simulink model "oUmControlador1"  (R2018a)
settings: Solver=VariableStepAuto  StartTime=0.0  StopTime=1000  RelTol=1e-3
settings Model: Creator=vittorfp  LastModifiedBy=vittorfp

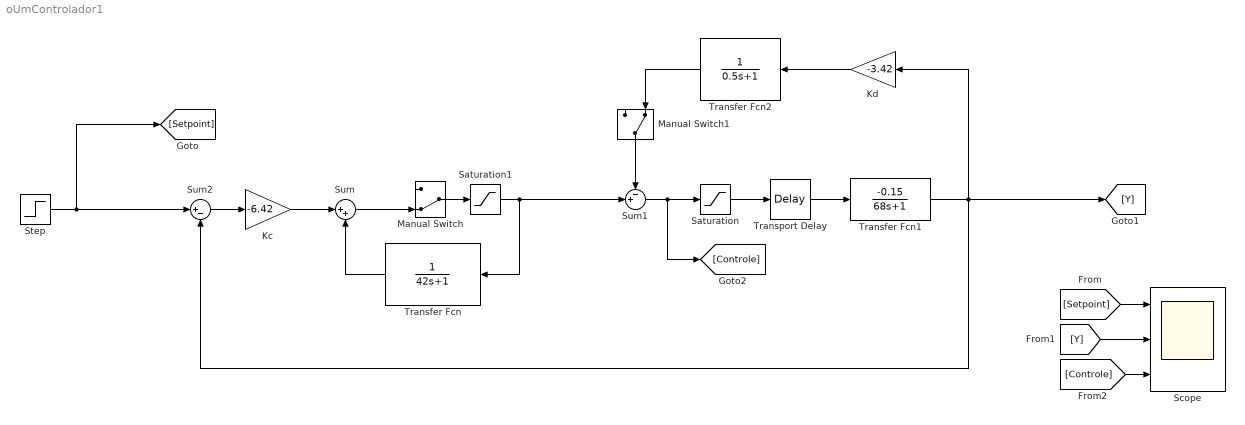
== system oUmControlador1 ==
  Kc : Gain  Gain=-6.42
  Kd : Gain  Gain=-3.42
  Manual Switch : ManualSwitch  CurrentSetting=0
  Manual Switch1 : ManualSwitch  CurrentSetting=0
  Saturation : Saturate  UpperLimit=10225  LowerLimit=-23200
  Saturation1 : Saturate  UpperLimit=10225  LowerLimit=-23200
  Scope : Scope  NumInputPorts=3
  Step : Step  After=2000  SampleTime=0
  Sum : Sum  Inputs=|++
  Sum1 : Sum  Inputs=-+|
  Sum2 : Sum  Inputs=|+-
  Transfer Fcn : TransferFcn  Denominator=[42 1]
  Transfer Fcn1 : TransferFcn  Numerator=[-0.15]  Denominator=[68 1]
  Transfer Fcn2 : TransferFcn  Denominator=[0.5 1]
  Transport Delay : TransportDelay  DelayTime=19
  wires:
  Kc/1 -> Sum/1
  Sum/1 -> Manual Switch/2
  Manual Switch/1 -> Saturation1/1
  Transfer Fcn/1 -> Sum/2
  Sum1/1 -> [Controle], Saturation/1
  Kd/1 -> Transfer Fcn2/1
  Transfer Fcn1/1 -> [Y], Kd/1, Sum2/2
  Sum2/1 -> Kc/1
  Step/1 -> Sum2/1, [Setpoint]
  Manual Switch1/1 -> Sum1/1
  Transfer Fcn2/1 -> Manual Switch1/2
  Saturation/1 -> Transport Delay/1
  Transport Delay/1 -> Transfer Fcn1/1
  [Setpoint] -> Scope/1
  [Y] -> Scope/2
  [Controle] -> Scope/3
  Saturation1/1 -> Sum1/2, Transfer Fcn/1
